simulink model "volo_agcdc_pipelined"  (R2012b)
settings: Solver=ode45  StartTime=0.0  StopTime=1000  RelTol=1e-3
PreLoadFcn:
  | volo_agcdc_init
InitFcn:
  | volo_agcdc_init
StartFcn:
  | volo_agcdc_init
values from neighbouring files (symbols this model uses):
  agc_idleState = 0    [volo_agcdc_init.m]
  agc_numAddrBits = agc_numOutputs + agc_numStateBits    [volo_agcdc_init.m]
  regDCRemoval_AvgLength = 64    [volo_agcdc_init.m]
  regSatDet_NumSamples = 16    [volo_agcdc_init.m]
undefined symbols (not defined in the file or in its folder): gcbh, xlBlockLoadCallback, xlGetNormalizedPeriod
libraries: xbsIndex_r4 x681, xbsEDKLib_r4 x1
(part 3 of 7)

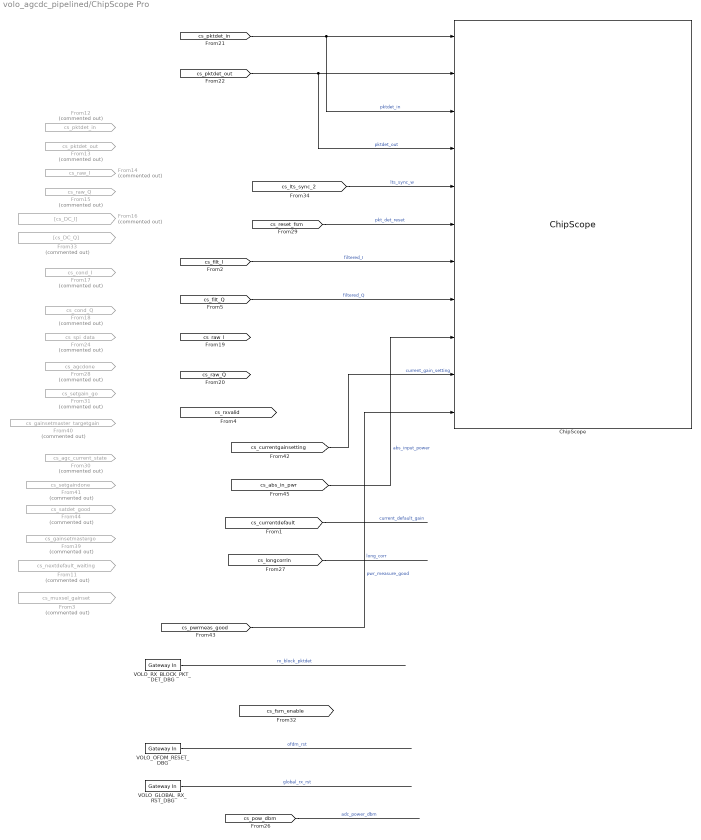
== system volo_agcdc_pipelined/ChipScope Pro ==
  ChipScope : xbsIndex_r4/ChipScope  num_trig_ports=2  current_port=0  show_trig_port=0  match_units=1  match_type=Basic  data_is_trigger=off  num_data_ports=9  data_depth=32768  SRL16s=on  add_bufg=on  match_type_t0=1  match_type_t1=1  match_type_t2=1  match_type_t3=1  match_type_t4=1  match_type_t5=1  match_type_t6=1  match_type_t7=1  match_type_t8=1  match_type_t9=1  match_type_t10=1  match_type_t11=1  match_type_t12=1  match_type_t13=1  match_type_t14=1  match_type_t15=1  match_units_t0=1  match_units_t1=1  match_units_t2=1  match_units_t3=1  match_units_t4=1  match_units_t5=1  match_units_t6=1  match_units_t7=1  match_units_t8=1  match_units_t9=1  match_units_t10=1  match_units_t11=1  match_units_t12=1  match_units_t13=1  match_units_t14=1  match_units_t15=1  dbl_ovrd=0  user_scan_chain=USER1  block_type=chipscope
      settings: infoedit="Enables run-time debugging and verification of signals by inserting ChipScope Pro ICON and ILA cores.<br><br>  Restrictions: <br>Only one ChipScope core can be instantiated in a System Generator design. A design or subsystem containing a ChipScope block must have at least one output port."
  From11 : From  Commented=on  GotoTag=cs_nextdefault_waiting  TagVisibility=global
  From12 : From  Commented=on  GotoTag=cs_pktdet_in  TagVisibility=global
  From13 : From  Commented=on  GotoTag=cs_pktdet_out  TagVisibility=global
  From14 : From  Commented=on  GotoTag=cs_raw_I  TagVisibility=global
  From15 : From  Commented=on  GotoTag=cs_raw_Q  TagVisibility=global
  From16 : From  Commented=on  GotoTag=cs_DC_I  TagVisibility=global
  From17 : From  Commented=on  GotoTag=cs_cond_I  TagVisibility=global
  From18 : From  Commented=on  GotoTag=cs_cond_Q  TagVisibility=global
  From24 : From  Commented=on  GotoTag=cs_spi_data  TagVisibility=global
  From28 : From  Commented=on  GotoTag=cs_agcdone  TagVisibility=global
  From3 : From  Commented=on  GotoTag=cs_muxsel_gainset  TagVisibility=global
  From30 : From  Commented=on  GotoTag=cs_agc_current_state  TagVisibility=global
  From31 : From  Commented=on  GotoTag=cs_setgain_go  TagVisibility=global
  From33 : From  Commented=on  GotoTag=cs_DC_Q  TagVisibility=global
  From39 : From  Commented=on  GotoTag=cs_gainsetmastergo  TagVisibility=global
  From40 : From  Commented=on  GotoTag=cs_gainsetmaster_targetgain  TagVisibility=global
  From41 : From  Commented=on  GotoTag=cs_setgaindone  TagVisibility=global
  From44 : From  Commented=on  GotoTag=cs_satdet_good  TagVisibility=global
  VOLO_GLOBAL_RX_RST_DBG : xbsIndex_r4/Gateway In  gui_display_data_type=Boolean  arith_type=Boolean  n_bits=32  bin_pt=0  preci_type=Single  exp_width=8  frac_width=24  quantization="Round  (unbiased: +/- Inf)"  overflow=Saturate  period=1  dbl_ovrd=off  timing_constraint=None  locs_specified=off  LOCs={}  UseAsADC=off  ADCChannel='1'  inherit_from_input=off  hdl_port=on  block_type=gatewayin
  VOLO_OFDM_RESET_DBG : xbsIndex_r4/Gateway In  gui_display_data_type=Boolean  arith_type=Boolean  n_bits=32  bin_pt=0  preci_type=Single  exp_width=8  frac_width=24  quantization="Round  (unbiased: +/- Inf)"  overflow=Saturate  period=1  dbl_ovrd=off  timing_constraint=None  locs_specified=off  LOCs={}  UseAsADC=off  ADCChannel='1'  inherit_from_input=off  hdl_port=on  block_type=gatewayin
  VOLO_RX_BLOCK_PKT_DET_DBG : xbsIndex_r4/Gateway In  gui_display_data_type=Boolean  arith_type=Boolean  n_bits=32  bin_pt=0  preci_type=Single  exp_width=8  frac_width=24  quantization="Round  (unbiased: +/- Inf)"  overflow=Saturate  period=1  dbl_ovrd=off  timing_constraint=None  locs_specified=off  LOCs={}  UseAsADC=off  ADCChannel='1'  inherit_from_input=off  hdl_port=on  block_type=gatewayin
  wires:
  [cs_pktdet_out] -> ChipScope/4, ChipScope/2  "pktdet_out"
  [cs_pktdet_in] -> ChipScope/3, ChipScope/1  "pktdet_in"
  [cs_lts_sync_2] -> ChipScope/5  "lts_sync_w"
  [cs_reset_fsm] -> ChipScope/6  "pkt_det_reset"
  VOLO_OFDM_RESET_DBG/1 -> ?  "ofdm_rst"
  VOLO_GLOBAL_RX_RST_DBG/1 -> ?  "global_rx_rst"
  VOLO_RX_BLOCK_PKT_DET_DBG/1 -> ?  "rx_block_pktdet"
  [cs_currentgainsetting] -> ChipScope/10  "current_gain_setting"
  [cs_pow_dbm] -> ?  "adc_power_dbm"
  [cs_abs_in_pwr] -> ChipScope/9  "abs_input_power"
  [cs_currentdefault] -> ?  "current_default_gain"
  [cs_longcorrin] -> ?  "long_corr"
  [cs_pwrmeas_good] -> ChipScope/11  "pwr_measure_good"
  [cs_filt_I] -> ChipScope/7  "filtered_I"
  [cs_filt_Q] -> ChipScope/8  "filtered_Q"

== system volo_agcdc_pipelined/Convert For WARPLab ==
  note: This maps [-127, 127] to [0, 255] while maintaining monotonicity.
  Fix9_0 : Inport
  AddSub : xbsIndex_r4/AddSub  mode=Addition  use_carryin=off  use_carryout=off  en=off  latency=0  precision=Full  arith_type=Unsigned  n_bits=16  bin_pt=14  quantization=Truncate  overflow=Wrap  dbl_ovrd=off  use_behavioral_HDL=off  hw_selection=Fabric  pipelined=off  block_type=addsub
  Constant : xbsIndex_r4/Constant  const=128  gui_display_data_type=Fixed-point  arith_type=Signed (2's comp)  n_bits=10  bin_pt=0  preci_type=Single  exp_width=8  frac_width=24  explicit_period=off  period=1  equ=P=C  opselect=C  inp2=PCIN>>17  opr=+  inp1=P  carry=CIN  dbl_ovrd=off  block_type=constant
  To_Fix10_0 : xbsIndex_r4/Convert  gui_display_data_type=Fixed-point  arith_type="Signed  (2's comp)"  n_bits=10  bin_pt=0  float_type=Single  exp_bits=8  fraction_bits=24  quantization=Truncate  overflow=Saturate  en=off  latency=0  dbl_ovrd=off  pipeline=off  block_type=convert
  To_Fix10_1 : xbsIndex_r4/Convert  gui_display_data_type=Fixed-point  arith_type=Unsigned  n_bits=10  bin_pt=0  float_type=Single  exp_bits=8  fraction_bits=24  quantization=Truncate  overflow=Saturate  en=off  latency=0  dbl_ovrd=off  pipeline=off  block_type=convert
  UFix10_0 : Outport
  wires:
  AddSub/1 -> To_Fix10_1/1
  Constant/1 -> AddSub/2
  To_Fix10_1/1 -> UFix10_0/1
  To_Fix10_0/1 -> AddSub/1
  Fix9_0/1 -> To_Fix10_0/1

== system volo_agcdc_pipelined/DC_REMOVAL ==
  note: Pipelined this logic REG
  note: ===== Revision History =====
      | 11_05_2013 - Updated to RxValid design for 80211, REG
      | 11_15_2013 - Added GainSetBusy reset to remove huge transition period
      | when AGC changes gains.
  note: This block latches the measured mean DC levels for I and Q when
      | the measurement good signal is high.
  Raw_I : Inport
  Raw_Q : Inport  Port=2
  RxValid : Inport  Port=3
  GainSetBusy : Inport  Port=4
  AddSub : xbsIndex_r4/AddSub  mode=Subtraction  use_carryin=off  use_carryout=off  en=off  latency=1  precision=User Defined  arith_type="Signed  (2's comp)"  n_bits=14  bin_pt=13  quantization=Truncate  overflow=Saturate  dbl_ovrd=off  use_behavioral_HDL=off  hw_selection=Fabric  pipelined=off  block_type=addsub
  AddSub1 : xbsIndex_r4/AddSub  mode=Subtraction  use_carryin=off  use_carryout=off  en=off  latency=1  precision=User Defined  arith_type="Signed  (2's comp)"  n_bits=14  bin_pt=13  quantization=Truncate  overflow=Saturate  dbl_ovrd=off  use_behavioral_HDL=off  hw_selection=Fabric  pipelined=off  block_type=addsub
  Binary Divide 128_1 : xbsIndex_r4/Shift  shift_dir=Right  shift_bits=6  en=off  latency=0  precision=User Defined  arith_type="Signed  (2's comp)"  n_bits=12  bin_pt=11  quantization=Truncate  overflow=Saturate  dbl_ovrd=off  block_type=shift
  Binary Divide 128_2 : xbsIndex_r4/Shift  shift_dir=Right  shift_bits=6  en=off  latency=0  precision=User Defined  arith_type="Signed  (2's comp)"  n_bits=12  bin_pt=11  quantization=Truncate  overflow=Saturate  dbl_ovrd=off  block_type=shift
  Convert3 : xbsIndex_r4/Convert  gui_display_data_type=Fixed-point  arith_type="Signed  (2's comp)"  n_bits=12  bin_pt=11  float_type=Single  exp_bits=8  fraction_bits=24  quantization="Round  (unbiased: Even Values)"  overflow=Saturate  en=off  latency=0  dbl_ovrd=off  pipeline=off  block_type=convert
  Convert4 : xbsIndex_r4/Convert  gui_display_data_type=Fixed-point  arith_type="Signed  (2's comp)"  n_bits=12  bin_pt=11  float_type=Single  exp_bits=8  fraction_bits=24  quantization="Round  (unbiased: Even Values)"  overflow=Saturate  en=off  latency=0  dbl_ovrd=off  pipeline=off  block_type=convert
  Delay{,1..3} (4 alike) : xbsIndex_r4/Delay  rst=off  infoeditControl=Selection of Reset will increase slice count due to use of real FFs and instead of SRLs  en=off  latency=1  dbl_ovrd=off  reg_retiming=off  block_type=delay
  Generate Reset : xbsIndex_r4/Logical  logical_function=AND  inputs=2  en=off  latency=0  precision=Full  arith_type=Unsigned  n_bits=16  bin_pt=0  align_bp=on  dbl_ovrd=off  block_type=logical
  Sliding Sum 64_1 : Subsystem
  Sliding Sum 64_2 : Subsystem
  To Register : xbsIndex_r4/To Register  shared_memory_name='regWSD_MeanDC_I'  init=0  ownership=Locally owned and initialized  explicit_data_type=on  gui_display_data_type=Fixed-point  arith_type="Signed  (2's comp)"  n_bits=12  bin_pt=11  preci_type=Single  dbl_ovrd=off  block_type=toreg
      settings: AttributesFormatString=<< %<shared_memory_name> >>  infoedit="Register block that writes data to a shared memory register.  Delay of one sample period."
  To Register1 : xbsIndex_r4/To Register  shared_memory_name='regWSD_MeanDC_Q'  init=0  ownership=Locally owned and initialized  explicit_data_type=on  gui_display_data_type=Fixed-point  arith_type="Signed  (2's comp)"  n_bits=12  bin_pt=11  preci_type=Single  dbl_ovrd=off  block_type=toreg
      settings: AttributesFormatString=<< %<shared_memory_name> >>  infoedit="Register block that writes data to a shared memory register.  Delay of one sample period."
  Valid Avg Counter : Subsystem
  Conditioned_I : Outport
  Conditioned_Q : Outport  Port=2
  MeanDC_Good : Outport  Port=3
  Rx_Valid_Out : Outport  Port=4
  tag scope: cs_cond_I=global, cs_cond_Q=global
  wires:
  Sliding Sum 64_1/1(Out) -> Binary Divide 128_1/1  "Sum Voltage"
  Raw_I/1 -> Sliding Sum 64_1/1(in), AddSub/1  "raw_I"
  Raw_Q/1 -> AddSub1/1, Sliding Sum 64_2/1(in)  "raw_Q"
  Generate Reset/1 -> Sliding Sum 64_1/2(rst), Sliding Sum 64_2/2(rst), Valid Avg Counter/2(RST)  "RST"
  Binary Divide 128_1/1 -> Delay/1, AddSub/2  "Mean I"
  Sliding Sum 64_2/1(Out) -> Binary Divide 128_2/1  "Sum Voltage"
  Binary Divide 128_2/1 -> Delay1/1, AddSub1/2  "Mean Q"
  AddSub1/1 -> Convert4/1, Conditioned_Q/1
  AddSub/1 -> Convert3/1, Conditioned_I/1
  RxValid/1 -> Delay3/1, Valid Avg Counter/1(RxValid), Sliding Sum 64_2/3(RxValid), Sliding Sum 64_1/3(RxValid)  "RxValid"
  GainSetBusy/1 -> Generate Reset/1
  [regAGC_GainSetResetsDCR_En] -> Generate Reset/2
  Convert3/1 -> [cs_cond_I]
  Convert4/1 -> [cs_cond_Q]
  Delay/1 -> To Register/1
  Delay1/1 -> To Register1/1
  Delay2/1 -> MeanDC_Good/1, To Register1/2, To Register/2
  Valid Avg Counter/1(DCMeas_Good) -> Delay2/1  "DC Output Good"
  Delay3/1 -> Rx_Valid_Out/1

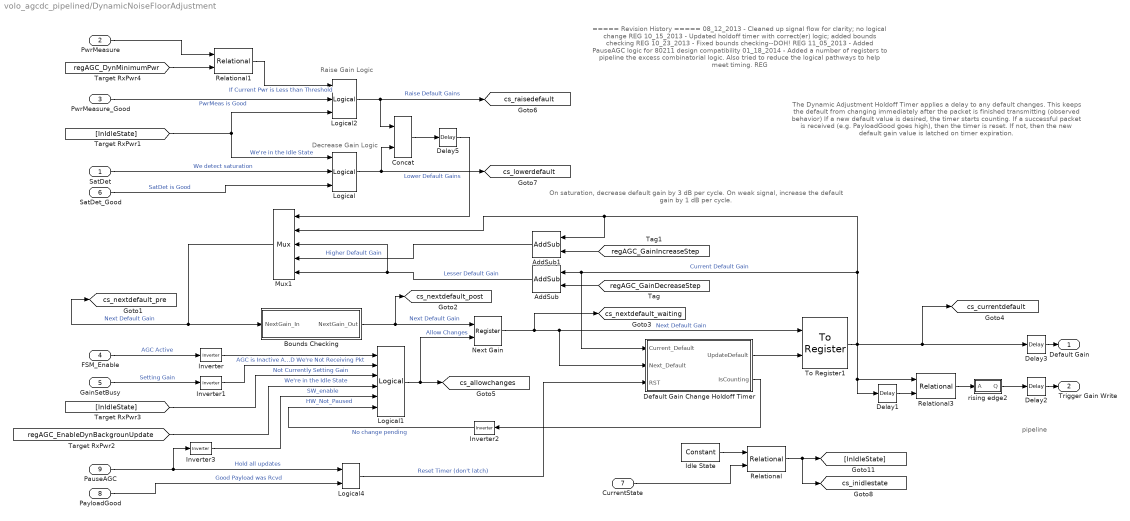
== system volo_agcdc_pipelined/DynamicNoiseFloorAdjustment ==
  note: pipeline
  note: ===== Revision History =====
      | 08_12_2013 - Cleaned up signal flow for clarity; no logical change REG
      | 10_15_2013 - Updated holdoff timer with correct(er) logic; added bounds checking REG
      | 10_23_2013 - Fixed bounds checking--DOH! REG
      | 11_05_2013 - Added PauseAGC logic for 80211 design compatibility
      | 01_18_2014 - Added a number of registers to pipeline the excess combinatorial logic. Also
      | tried to reduce the logical pathways to help meet timing. REG
  note: On saturation, decrease default gain by 3 dB per cycle.
      | On weak signal, increase the default gain by 1 dB per cycle.
  note: Decrease Gain Logic
  note: Raise Gain Logic
  note: The Dynamic Adjustment Holdoff Timer applies a delay to any default changes.
      | This keeps the default from changing immediately after the packet is finished transmitting (observed behavior)
      |  If a new default value is desired, the timer starts counting.
      | If a successful packet is received (e.g. PayloadGood goes high), then the timer
      | is reset. If not, then the new default gain value is latched on timer expiration.
  SatDet : Inport
  PwrMeasure : Inport  Port=2
  PwrMeasure_Good : Inport  Port=3
  FSM_Enable : Inport  Port=4
  GainSetBusy : Inport  Port=5
  SatDet_Good : Inport  Port=6
  CurrentState : Inport  Port=7
  PayloadGood : Inport  Port=8
  PauseAGC : Inport  Port=9
  AddSub : xbsIndex_r4/AddSub  mode=Subtraction  use_carryin=off  use_carryout=off  en=off  latency=0  precision=User Defined  arith_type=Unsigned  n_bits=6  bin_pt=0  quantization=Truncate  overflow=Saturate  dbl_ovrd=off  use_behavioral_HDL=off  hw_selection=Fabric  pipelined=off  block_type=addsub
  AddSub1 : xbsIndex_r4/AddSub  mode=Addition  use_carryin=off  use_carryout=off  en=off  latency=0  precision=User Defined  arith_type=Unsigned  n_bits=6  bin_pt=0  quantization=Truncate  overflow=Saturate  dbl_ovrd=off  use_behavioral_HDL=off  hw_selection=Fabric  pipelined=off  block_type=addsub
  Bounds Checking : Subsystem
  Concat : xbsIndex_r4/Concat  num_inputs=2  dbl_ovrd=off  block_type=concat
  Default Gain Change Holdoff Timer : Subsystem
  Delay1 : xbsIndex_r4/Delay  rst=off  infoeditControl=Selection of Reset will increase slice count due to use of real FFs and instead of SRLs  en=off  latency=1  dbl_ovrd=off  reg_retiming=off  block_type=delay
  Delay2 : xbsIndex_r4/Delay  rst=off  infoeditControl=Selection of Reset will increase slice count due to use of real FFs and instead of SRLs  en=off  latency=4  dbl_ovrd=off  reg_retiming=off  block_type=delay
  Delay3 : xbsIndex_r4/Delay  rst=off  infoeditControl=Selection of Reset will increase slice count due to use of real FFs and instead of SRLs  en=off  latency=4  dbl_ovrd=off  reg_retiming=off  block_type=delay
  Delay5 : xbsIndex_r4/Delay  rst=off  infoeditControl=Selection of Reset will increase slice count due to use of real FFs and instead of SRLs  en=off  latency=1  dbl_ovrd=off  reg_retiming=off  block_type=delay
  Idle State : xbsIndex_r4/Constant  const=0  gui_display_data_type=Fixed-point  arith_type=Unsigned  n_bits=3  bin_pt=0  preci_type=Single  exp_width=8  frac_width=24  explicit_period=off  period=1  equ=P=C  opselect=C  inp2=PCIN>>17  opr=+  inp1=P  carry=CIN  dbl_ovrd=off  block_type=constant
  Inverter{,1..3} (4 alike) : xbsIndex_r4/Inverter  en=off  latency=0  dbl_ovrd=off  block_type=inv
  Logical : xbsIndex_r4/Logical  logical_function=AND  inputs=3  en=off  latency=0  precision=Full  arith_type=Unsigned  n_bits=16  bin_pt=0  align_bp=on  dbl_ovrd=off  block_type=logical
  Logical1 : xbsIndex_r4/Logical  logical_function=AND  inputs=6  en=off  latency=0  precision=Full  arith_type=Unsigned  n_bits=16  bin_pt=0  align_bp=on  dbl_ovrd=off  block_type=logical
  Logical2 : xbsIndex_r4/Logical  logical_function=AND  inputs=3  en=off  latency=0  precision=Full  arith_type=Unsigned  n_bits=16  bin_pt=0  align_bp=on  dbl_ovrd=off  block_type=logical
  Logical4 : xbsIndex_r4/Logical  logical_function=OR  inputs=2  en=off  latency=0  precision=Full  arith_type=Unsigned  n_bits=16  bin_pt=0  align_bp=on  dbl_ovrd=off  block_type=logical
  Mux1 : xbsIndex_r4/Mux  inputs=4  en=off  latency=0  precision=Full  arith_type=Unsigned  n_bits=16  bin_pt=14  quantization=Truncate  overflow=Wrap  dbl_ovrd=off  block_type=mux
  Next Gain : xbsIndex_r4/Register  init=0  rst=off  en=on  dbl_ovrd=off  block_type=register
  Relational : xbsIndex_r4/Relational  mode=a=b  en=off  latency=0  dbl_ovrd=off  block_type=relational
  Relational1 : xbsIndex_r4/Relational  mode=a<b  en=off  latency=0  dbl_ovrd=off  block_type=relational
  Relational3 : xbsIndex_r4/Relational  mode=a!=b  en=off  latency=0  dbl_ovrd=off  block_type=relational
  To Register1 : xbsIndex_r4/To Register  shared_memory_name='regWSD_DynDefaultGain'  init=0  ownership=Locally owned and initialized  explicit_data_type=on  gui_display_data_type=Fixed-point  arith_type=Unsigned  n_bits=6  bin_pt=0  preci_type=Single  dbl_ovrd=off  block_type=toreg
      settings: AttributesFormatString=<< %<shared_memory_name> >>  infoedit="Register block that writes data to a shared memory register.  Delay of one sample period."
  rising edge2 : Subsystem
  Default Gain : Outport
  Trigger Gain Write : Outport  Port=2
  tag scope: cs_allowchanges=global, cs_currentdefault=global, cs_inidlestate=global, cs_lowerdefault=global, cs_nextdefault_post=global, cs_nextdefault_pre=global, cs_nextdefault_waiting=global, cs_raisedefault=global
  wires:
  Next Gain/1 -> [cs_nextdefault_waiting], Default Gain Change Holdoff Timer/2(Next_Default), To Register1/1  "Next Default Gain"
  AddSub/1 -> Mux1/5, Mux1/3  "Lesser Default Gain"
  SatDet/1 -> Logical/2  "We detect saturation"
  Logical/1 -> [cs_lowerdefault], Concat/2  "Lower Default Gains"
  Mux1/1 -> Bounds Checking/1(NextGain_In), [cs_nextdefault_pre]  "Next Default Gain"
  [regAGC_GainIncreaseStep] -> AddSub1/2
  [regAGC_GainDecreaseStep] -> AddSub/2
  FSM_Enable/1 -> Inverter/1  "AGC Active"
  Inverter/1 -> Logical1/1  "AGC is Inactive AND We're Not Receiving Pkt"
  Logical1/1 -> Next Gain/2, [cs_allowchanges]  "Allow Changes"
  AddSub1/1 -> Mux1/4  "Higher Default Gain"
  SatDet_Good/1 -> Logical/3  "SatDet is Good"
  PwrMeasure/1 -> Relational1/1
  [regAGC_DynMinimumPwr] -> Relational1/2
  Relational1/1 -> Logical2/1  "If Current Pwr is Less than Threshold"
  PwrMeasure_Good/1 -> Logical2/2  "PwrMeas is Good"
  Idle State/1 -> Relational/1
  CurrentState/1 -> Relational/2
  Relational/1 -> [cs_inidlestate], [InIdleState]
  [InIdleState] -> Logical/1, Logical2/3  "We're in the Idle State"
  GainSetBusy/1 -> Inverter1/1  "Setting Gain"
  Inverter1/1 -> Logical1/2  "Not Currently Setting Gain"
  Logical2/1 -> [cs_raisedefault], Concat/1  "Raise Default Gains"
  [InIdleState] -> Logical1/3  "We're in the Idle State"
  To Register1/1 -> Delay1/1, Relational3/1, [cs_currentdefault], Delay3/1, Default Gain Change Holdoff Timer/1(Current_Default), AddSub/1, Mux1/2, AddSub1/1  "Current Default Gain"
  Delay1/1 -> Relational3/2
  rising edge2/1(Q) -> Delay2/1
  Relational3/1 -> rising edge2/1(A)
  PayloadGood/1 -> Logical4/2  "Good Payload was Rcvd"
  Default Gain Change Holdoff Timer/1(UpdateDefault) -> To Register1/2
  Bounds Checking/1(NextGain_Out) -> [cs_nextdefault_post], Next Gain/1  "Next Default Gain"
  [regAGC_EnableDynBackgrounUpdate] -> Logical1/4  "SW_enable"
  PauseAGC/1 -> Inverter3/1, Logical4/1  "Hold all updates"
  Inverter3/1 -> Logical1/5  "HW_Not_Paused"
  Logical4/1 -> Default Gain Change Holdoff Timer/3(RST)  "Reset Timer (don't latch)"
  Default Gain Change Holdoff Timer/2(IsCounting) -> Inverter2/1
  Inverter2/1 -> Logical1/6  "No change pending"
  Delay3/1 -> Default Gain/1
  Delay2/1 -> Trigger Gain Write/1
  Delay5/1 -> Mux1/1
  Concat/1 -> Delay5/1
